simulink model "SecRwLtStArmScrnTrgtPosSelc"  (R2018b)
settings: Solver=FixedStepDiscrete  StartTime=0.0  StopTime=10.0  FixedStep=0.01  RelTol=1e-3
undefined symbols (not defined in the file or in its folder): KeSMSw6sAcsEntrySecRwLtStArmScrnPos_Val, KeSMSw6sAcsEntrySecRwLtStArmScrnPosMax_Val, KeSMSw6sAcsEntrySecRwLtStArmScrnPosMin_Val, KeSMSw6sAcsExtSecRwLtStArmScrnPos_Val, KeSMSw6sAcsExtSecRwLtStArmScrnPosMax_Val, KeSMSw6sAcsExtSecRwLtStArmScrnPosMin_Val, KeSMSwAcsEntrySecRwLtStArmScrnPos_Val, KeSMSwAcsEntrySecRwLtStArmScrnPosMax_Val, KeSMSwAcsEntrySecRwLtStArmScrnPosMin_Val, KeSMSwAcsExtSecRwLtStArmScrnPos_Val, KeSMSwAcsExtSecRwLtStArmScrnPosMax_Val, KeSMSwAcsExtSecRwLtStArmScrnPosMin_Val
libraries: TrgtPosSelcLib x3
settings Model: Creator=sn2xws  LastModifiedBy=sn2xws
settings DataIOCC: SaveFormat=StructureWithTime
settings OptimizationCC: DefaultParameterBehavior=Inlined  EnhancedBackFolding=on  PassReuseOutputArgsAs=Individual arguments  ZeroExternalMemoryAtStartup=off  ZeroInternalMemoryAtStartup=off  OptimizeBlockOrder=speed  DifferentSizesBufferReuse=on  OptimizationCustomize=off
settings DebuggingCC: ParameterTunabilityLossMsg=error
settings ModelReferenceCC: ModelReferenceNumInstancesAllowed=Single
settings SFSimCC: MATLABDynamicMemAlloc=off
settings RTWCC: SystemTargetFile=autosar.tlc  GenCodeOnly=on  TemplateMakefile=ert_default_tmf  Description=AUTOSAR  GenerateReport=on  IncludeHyperlinkInReport=on  LaunchReport=on  GenerateTraceInfo=on  GenerateTraceReport=on  GenerateTraceReportSl=on  GenerateTraceReportSf=on  GenerateTraceReportEml=on  GenerateCodeMetricsReport=on
settings CodeAppCC: ForceParamTrailComments=on  IgnoreCustomStorageClasses=off  OperatorAnnotations=on  SimulinkDataObjDesc=on  SFDataObjDesc=on  InsertBlockDesc=on
settings STFCustomTargetCC: TargetLangStandard=C99 (ISO)  MultiwordLength=256  ParMdlRefBuildCompliant=on  CompOptLevelCompliant=on  IncludeMdlTerminateFcn=off  CombineOutputUpdateFcns=on  SuppressErrorStatus=on  ERTCustomFileBanners=on  SupportNonFinite=off  SupportComplex=off  SupportContinuousTime=off  SupportNonInlinedSFcns=off  RemoveResetFunc=on  MATLABClassNameForMDSCustomization=Simulink.SoftwareTarget.ERTCustomization  AutosarCompliant=on  UseToolchainInfoCompliant=on  LookupTableObjectStructAxisOrder=2,1,3,4,...  LUTObjectStructOrderEvenSpacing=Size,Table,Breakpoints  SystemTargetFile=autosar.tlc
settings ERTTargetCC: TargetLangStandard=C99 (ISO)  ConcurrentExecutionCompliant=off  IncludeMdlTerminateFcn=off  SuppressErrorStatus=on  SupportNonFinite=off  SupportComplex=off  ModelStepFunctionPrototypeControlCompliant=off  CPPClassGenCompliant=off  AutosarCompliant=on  LookupTableObjectStructAxisOrder=2,1,3,4,...  LUTObjectStructOrderEvenSpacing=Size,Table,Breakpoints  InlinedParameterPlacement=NonHierarchical  ERTCustomFileTemplate=example_file_process.tlc  ERTFilePackagingFormat=Compact

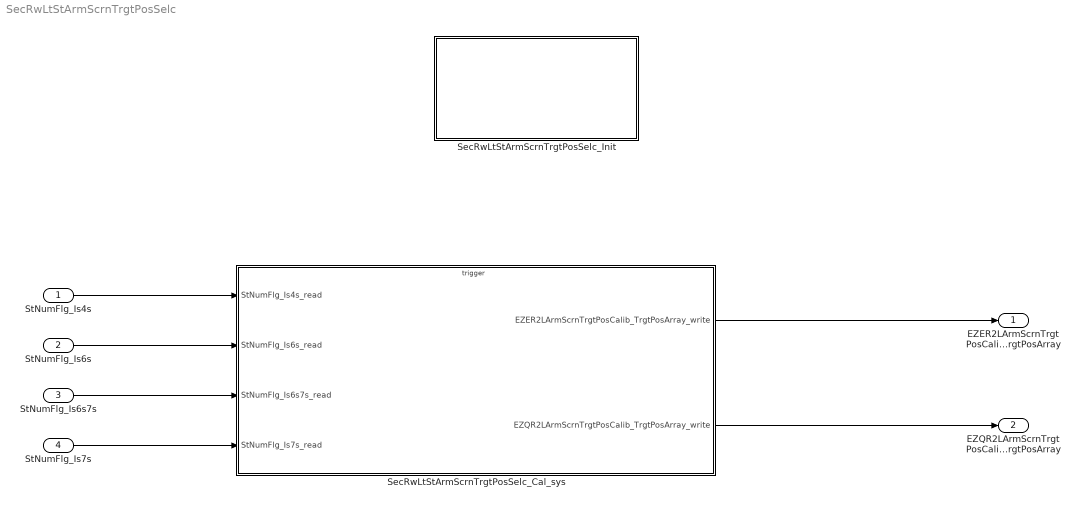
== system SecRwLtStArmScrnTrgtPosSelc ==
  StNumFlg_Is4s : Inport  OutDataTypeStr=boolean  PortDimensions=1
  StNumFlg_Is6s : Inport  Port=2  OutDataTypeStr=boolean  PortDimensions=1
  StNumFlg_Is6s7s : Inport  Port=3  OutDataTypeStr=boolean  PortDimensions=1
  StNumFlg_Is7s : Inport  Port=4  OutDataTypeStr=boolean  PortDimensions=1
  SecRwLtStArmScrnTrgtPosSelc_Cal_sys : Subsystem
  SecRwLtStArmScrnTrgtPosSelc_Init : Subsystem
  EZER2LArmScrnTrgtPosCalib_TrgtPosArray : Outport  Description=|  OutDataTypeStr=uint16  PortDimensions=3
      | 0:Pos
      | 1:Max
      | 2:Min
  EZQR2LArmScrnTrgtPosCalib_TrgtPosArray : Outport  Description=|  Port=2  OutDataTypeStr=uint16  PortDimensions=3
      | 0:Pos
      | 1:Max
      | 2:Min
  wires:
  StNumFlg_Is4s/1 -> SecRwLtStArmScrnTrgtPosSelc_Cal_sys/1(StNumFlg_Is4s_read)
  StNumFlg_Is6s/1 -> SecRwLtStArmScrnTrgtPosSelc_Cal_sys/2(StNumFlg_Is6s_read)
  StNumFlg_Is6s7s/1 -> SecRwLtStArmScrnTrgtPosSelc_Cal_sys/3(StNumFlg_Is6s7s_read)
  StNumFlg_Is7s/1 -> SecRwLtStArmScrnTrgtPosSelc_Cal_sys/4(StNumFlg_Is7s_read)
  SecRwLtStArmScrnTrgtPosSelc_Cal_sys/1(EZER2LArmScrnTrgtPosCalib_TrgtPosArray_write) -> EZER2LArmScrnTrgtPosCalib_TrgtPosArray/1
  SecRwLtStArmScrnTrgtPosSelc_Cal_sys/2(EZQR2LArmScrnTrgtPosCalib_TrgtPosArray_write) -> EZQR2LArmScrnTrgtPosCalib_TrgtPosArray/1

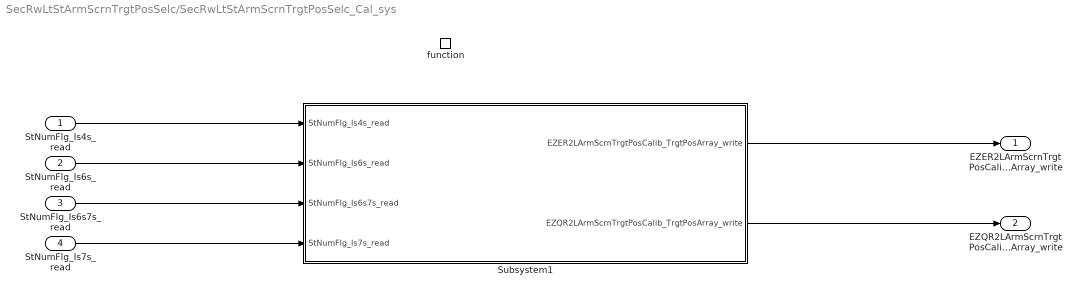
== system SecRwLtStArmScrnTrgtPosSelc/SecRwLtStArmScrnTrgtPosSelc_Cal_sys ==
  StNumFlg_Is4s_read : Inport
  StNumFlg_Is6s_read : Inport  Port=2
  StNumFlg_Is6s7s_read : Inport  Port=3
  StNumFlg_Is7s_read : Inport  Port=4
  function : TriggerPort  TriggerType=function-call  IsSimulinkFunction=on  FunctionName=SecRwLtStArmScrnTrgtPosSelc_Cal  VariantControl=(inherit)
  Subsystem1 : Subsystem
  EZER2LArmScrnTrgtPosCalib_TrgtPosArray_write : Outport
      settings: EnsureOutportIsVirtual=on
  EZQR2LArmScrnTrgtPosCalib_TrgtPosArray_write : Outport  Port=2
      settings: EnsureOutportIsVirtual=on
  wires:
  Subsystem1/1(EZER2LArmScrnTrgtPosCalib_TrgtPosArray_write) -> EZER2LArmScrnTrgtPosCalib_TrgtPosArray_write/1
  Subsystem1/2(EZQR2LArmScrnTrgtPosCalib_TrgtPosArray_write) -> EZQR2LArmScrnTrgtPosCalib_TrgtPosArray_write/1
  StNumFlg_Is4s_read/1 -> Subsystem1/1(StNumFlg_Is4s_read)
  StNumFlg_Is6s_read/1 -> Subsystem1/2(StNumFlg_Is6s_read)
  StNumFlg_Is6s7s_read/1 -> Subsystem1/3(StNumFlg_Is6s7s_read)
  StNumFlg_Is7s_read/1 -> Subsystem1/4(StNumFlg_Is7s_read)

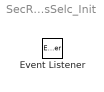
== system SecRwLtStArmScrnTrgtPosSelc/SecRwLtStArmScrnTrgtPosSelc_Init ==
  Event Listener : EventListener  EventName=reset

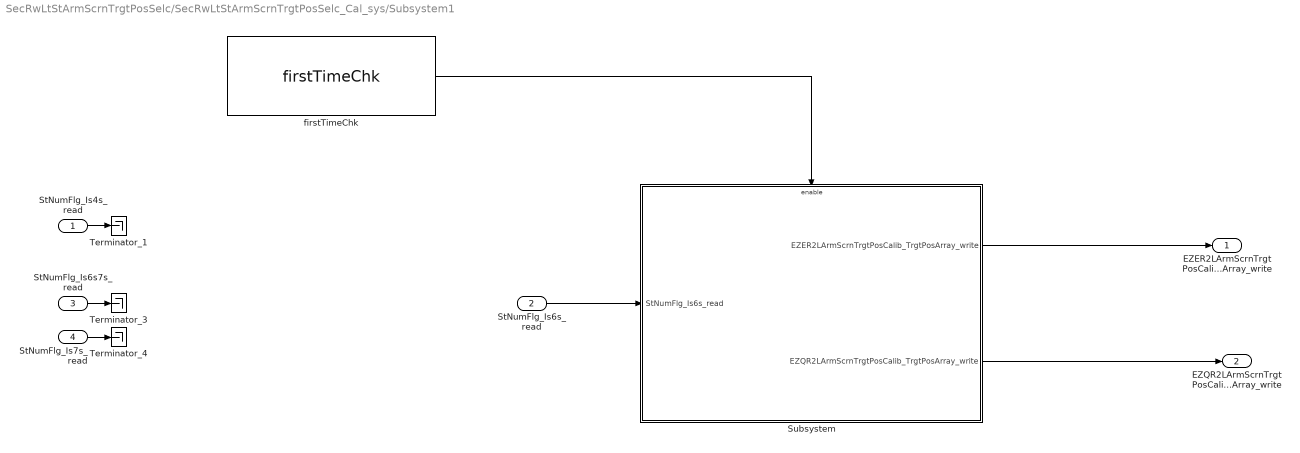
== system SecRwLtStArmScrnTrgtPosSelc/SecRwLtStArmScrnTrgtPosSelc_Cal_sys/Subsystem1 ==
  StNumFlg_Is4s_read : Inport
  StNumFlg_Is6s_read : Inport  Port=2
  StNumFlg_Is6s7s_read : Inport  Port=3
  StNumFlg_Is7s_read : Inport  Port=4
  Subsystem : Subsystem
  Terminator_1 : Terminator
  Terminator_3 : Terminator
  Terminator_4 : Terminator
  firstTimeChk : TrgtPosSelcLib/firstTimeChk  SystemSampleTime=-1
  EZER2LArmScrnTrgtPosCalib_TrgtPosArray_write : Outport
      settings: EnsureOutportIsVirtual=on
  EZQR2LArmScrnTrgtPosCalib_TrgtPosArray_write : Outport  Port=2
      settings: EnsureOutportIsVirtual=on
  wires:
  StNumFlg_Is6s_read/1 -> Subsystem/1(StNumFlg_Is6s_read)
  StNumFlg_Is4s_read/1 -> Terminator_1/1
  Subsystem/1(EZER2LArmScrnTrgtPosCalib_TrgtPosArray_write) -> EZER2LArmScrnTrgtPosCalib_TrgtPosArray_write/1
  StNumFlg_Is6s7s_read/1 -> Terminator_3/1
  Subsystem/2(EZQR2LArmScrnTrgtPosCalib_TrgtPosArray_write) -> EZQR2LArmScrnTrgtPosCalib_TrgtPosArray_write/1
  StNumFlg_Is7s_read/1 -> Terminator_4/1
  firstTimeChk/1 -> Subsystem/Enable

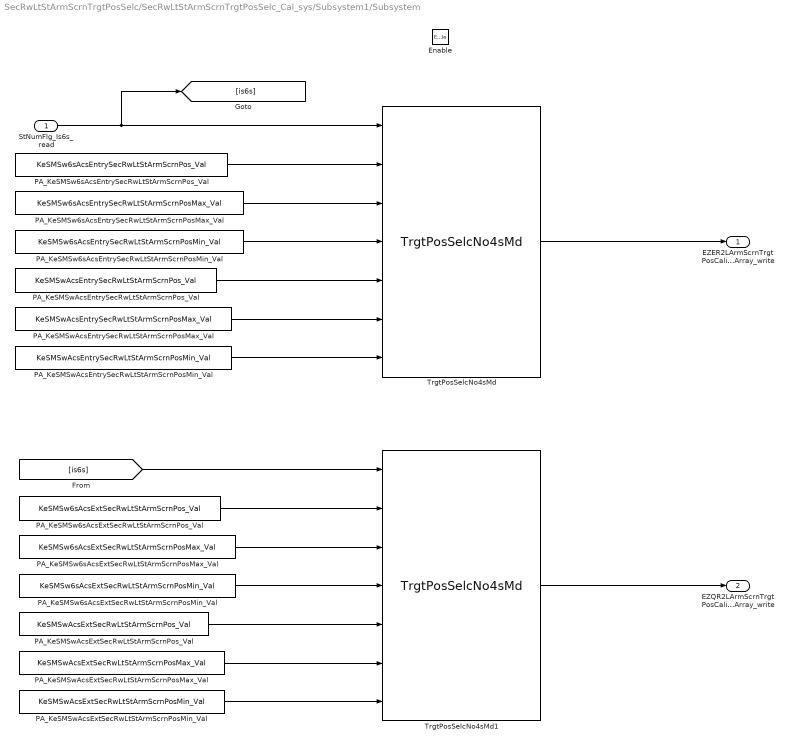
== system SecRwLtStArmScrnTrgtPosSelc/SecRwLtStArmScrnTrgtPosSelc_Cal_sys/Subsystem1/Subsystem ==
  StNumFlg_Is6s_read : Inport
  Enable : EnablePort
  PA_KeSMSw6sAcsEntrySecRwLtStArmScrnPosMax_Val : Constant  Value=KeSMSw6sAcsEntrySecRwLtStArmScrnPosMax_Val
  PA_KeSMSw6sAcsEntrySecRwLtStArmScrnPosMin_Val : Constant  Value=KeSMSw6sAcsEntrySecRwLtStArmScrnPosMin_Val
  PA_KeSMSw6sAcsEntrySecRwLtStArmScrnPos_Val : Constant  Value=KeSMSw6sAcsEntrySecRwLtStArmScrnPos_Val
  PA_KeSMSw6sAcsExtSecRwLtStArmScrnPosMax_Val : Constant  Value=KeSMSw6sAcsExtSecRwLtStArmScrnPosMax_Val
  PA_KeSMSw6sAcsExtSecRwLtStArmScrnPosMin_Val : Constant  Value=KeSMSw6sAcsExtSecRwLtStArmScrnPosMin_Val
  PA_KeSMSw6sAcsExtSecRwLtStArmScrnPos_Val : Constant  Value=KeSMSw6sAcsExtSecRwLtStArmScrnPos_Val
  PA_KeSMSwAcsEntrySecRwLtStArmScrnPosMax_Val : Constant  Value=KeSMSwAcsEntrySecRwLtStArmScrnPosMax_Val
  PA_KeSMSwAcsEntrySecRwLtStArmScrnPosMin_Val : Constant  Value=KeSMSwAcsEntrySecRwLtStArmScrnPosMin_Val
  PA_KeSMSwAcsEntrySecRwLtStArmScrnPos_Val : Constant  Value=KeSMSwAcsEntrySecRwLtStArmScrnPos_Val
  PA_KeSMSwAcsExtSecRwLtStArmScrnPosMax_Val : Constant  Value=KeSMSwAcsExtSecRwLtStArmScrnPosMax_Val
  PA_KeSMSwAcsExtSecRwLtStArmScrnPosMin_Val : Constant  Value=KeSMSwAcsExtSecRwLtStArmScrnPosMin_Val
  PA_KeSMSwAcsExtSecRwLtStArmScrnPos_Val : Constant  Value=KeSMSwAcsExtSecRwLtStArmScrnPos_Val
  TrgtPosSelcNo4sMd : TrgtPosSelcLib/TrgtPosSelcNo4sMd  SystemSampleTime=-1
  TrgtPosSelcNo4sMd1 : TrgtPosSelcLib/TrgtPosSelcNo4sMd  SystemSampleTime=-1
  EZER2LArmScrnTrgtPosCalib_TrgtPosArray_write : Outport
      settings: EnsureOutportIsVirtual=on
  EZQR2LArmScrnTrgtPosCalib_TrgtPosArray_write : Outport  Port=2
      settings: EnsureOutportIsVirtual=on
  wires:
  PA_KeSMSwAcsEntrySecRwLtStArmScrnPosMin_Val/1 -> TrgtPosSelcNo4sMd/7
  PA_KeSMSw6sAcsEntrySecRwLtStArmScrnPosMin_Val/1 -> TrgtPosSelcNo4sMd/4
  PA_KeSMSwAcsEntrySecRwLtStArmScrnPos_Val/1 -> TrgtPosSelcNo4sMd/5
  PA_KeSMSw6sAcsEntrySecRwLtStArmScrnPos_Val/1 -> TrgtPosSelcNo4sMd/2
  StNumFlg_Is6s_read/1 -> [is6s], TrgtPosSelcNo4sMd/1
  PA_KeSMSwAcsExtSecRwLtStArmScrnPosMin_Val/1 -> TrgtPosSelcNo4sMd1/7
  PA_KeSMSwAcsExtSecRwLtStArmScrnPosMax_Val/1 -> TrgtPosSelcNo4sMd1/6
  PA_KeSMSwAcsEntrySecRwLtStArmScrnPosMax_Val/1 -> TrgtPosSelcNo4sMd/6
  PA_KeSMSw6sAcsExtSecRwLtStArmScrnPosMax_Val/1 -> TrgtPosSelcNo4sMd1/3
  PA_KeSMSw6sAcsEntrySecRwLtStArmScrnPosMax_Val/1 -> TrgtPosSelcNo4sMd/3
  PA_KeSMSwAcsExtSecRwLtStArmScrnPos_Val/1 -> TrgtPosSelcNo4sMd1/5
  PA_KeSMSw6sAcsExtSecRwLtStArmScrnPosMin_Val/1 -> TrgtPosSelcNo4sMd1/4
  TrgtPosSelcNo4sMd/1 -> EZER2LArmScrnTrgtPosCalib_TrgtPosArray_write/1
  TrgtPosSelcNo4sMd1/1 -> EZQR2LArmScrnTrgtPosCalib_TrgtPosArray_write/1
  PA_KeSMSw6sAcsExtSecRwLtStArmScrnPos_Val/1 -> TrgtPosSelcNo4sMd1/2
  [is6s] -> TrgtPosSelcNo4sMd1/1
